simulink subsystem "Motor_Control_Feedback"  (R2024a)
settings: Solver=VariableStepAuto  StartTime=0.0  StopTime=10.0  RelTol=1e-3
undefined symbols (not defined in the file or in its folder): MaxMotorVoltage, motorFBRate, wToVolt
settings Model: Creator=Peter  LastModifiedBy=Peter

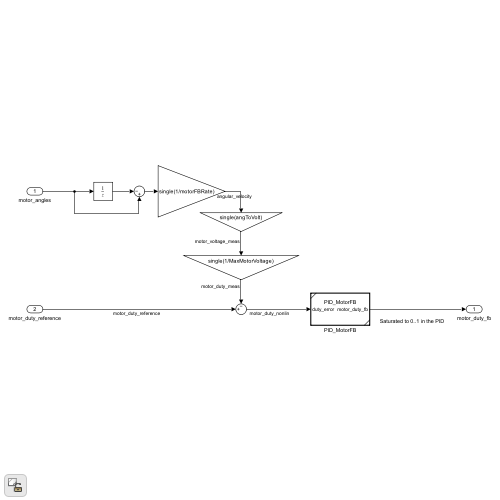
[thumbnail: Simulink's stored preview of the top-level diagram]
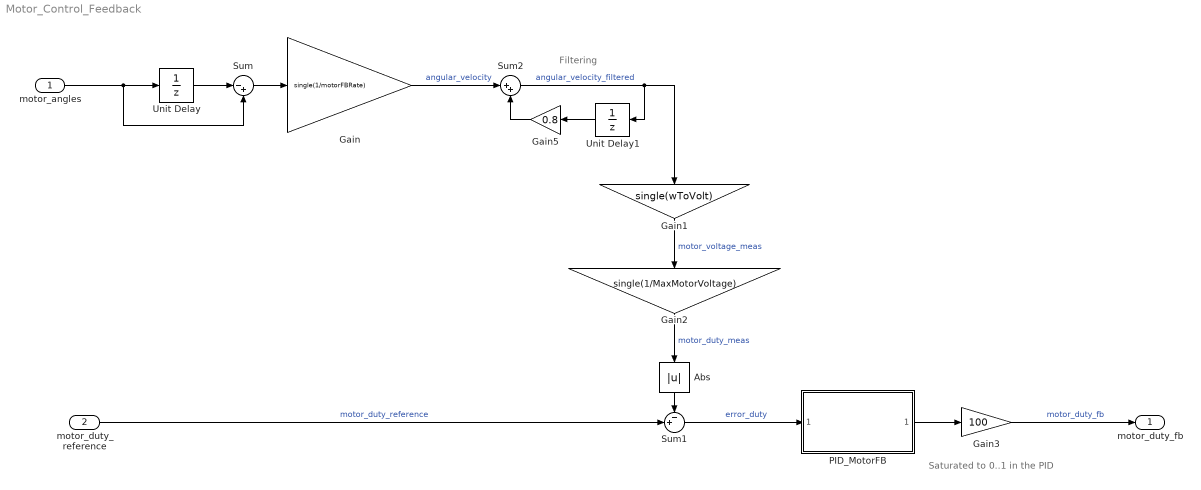
== system Motor_Control_Feedback ==
  note: Saturated to 0..1 in the PID
  note: Filtering
  motor_angles : Inport
  motor_duty_reference : Inport  Port=2
  Abs : Abs  SaturateOnIntegerOverflow=off
  Gain : Gain  Gain=single(1/motorFBRate)
  Gain1 : Gain  Gain=single(wToVolt)  OutDataTypeStr=single
  Gain2 : Gain  Gain=single(1/MaxMotorVoltage)
  Gain3 : Gain  Gain=100
  Gain5 : Gain  Gain=0.8
  PID_MotorFB : Subsystem  TreatAsAtomicUnit=on  SystemSampleTime=motorFBRate  ReferencedSubsystem=PID_MotorFB
  Sum : Sum  Inputs=|-+
  Sum1 : Sum  Inputs=-+|
  Sum2 : Sum  Inputs=|++
  Unit Delay : UnitDelay  SampleTime=motorFBRate  HasFrameUpgradeWarning=on
  Unit Delay1 : UnitDelay  SampleTime=motorFBRate  HasFrameUpgradeWarning=on
  motor_duty_fb : Outport
  wires:
  Sum1/1 -> PID_MotorFB/1  "error_duty"
  motor_angles/1 -> Unit Delay/1, Sum/2
  motor_duty_reference/1 -> Sum1/2  "motor_duty_reference"
  Unit Delay/1 -> Sum/1
  Sum/1 -> Gain/1
  Gain/1 -> Sum2/1  "angular_velocity"
  Gain1/1 -> Gain2/1  "motor_voltage_meas"
  Gain2/1 -> Abs/1  "motor_duty_meas"
  PID_MotorFB/1 -> Gain3/1
  Gain3/1 -> motor_duty_fb/1  "motor_duty_fb"
  Abs/1 -> Sum1/1
  Gain5/1 -> Sum2/2
  Sum2/1 -> Unit Delay1/1, Gain1/1  "angular_velocity_filtered"
  Unit Delay1/1 -> Gain5/1
